simulink model "wind_model"  (R2021b)
settings: Solver=VariableStepAuto  StartTime=0.0  StopTime=500  RelTol=1e-3
values from neighbouring files (symbols this model uses):
  F = 0.0555 * (1+8*a_bar^2)*t^2*b^3    [ImIiCompute.m]
  r = 1000    [MPC.m]
undefined symbols (not defined in the file or in its folder): Light, MIL
libraries: aerolibwind2 x2, simulink x1
settings Model: Creator=zhongyuliang  LastModifiedBy=zhongyuliang

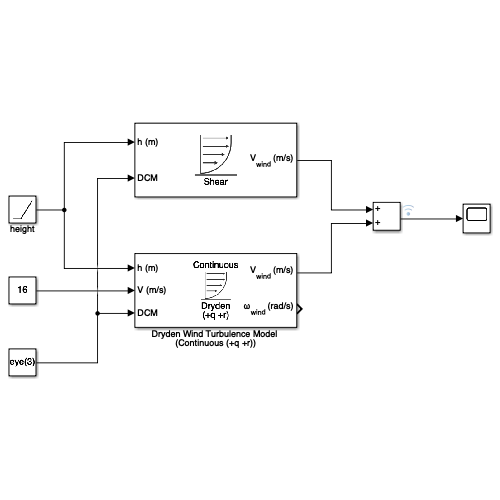
[thumbnail: Simulink's stored preview of the top-level diagram]
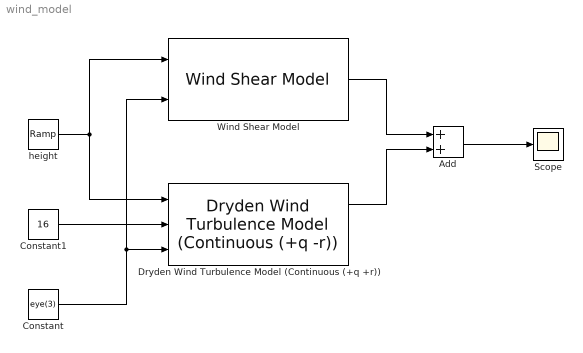
== system wind_model ==
  Add : Sum
  Constant : Constant  Value=eye(3)
  Constant1 : Constant  Value=16
  Dryden Wind Turbulence Model (Continuous (+q +r)) : aerolibwind2/Dryden Wind Turbulence Model  (Continuous (+q -r))  units=Metric (MKS)  spec=MIL-F-8785C  model=Continuous Dryden (+q +r)  W20=3  Wdeg=0  TurbProb=10^-2 - Light  L_high=533.4  Wingspan=10  ts=0.1  Seed=[23341 23342 23343 23344]  T_on=on
  Scope : Scope
  Wind Shear Model : aerolibwind2/Wind Shear Model  units=Metric (MKS)  phase=Category C - Terminal Flight Phase  W_20=15  Wdeg=0
  height : simulink/Sources/Ramp  slope=1  start=0  InitialOutput=0
  wires:
  Constant/1 -> Wind Shear Model/2, Dryden Wind Turbulence Model (Continuous (+q +r))/3
  height/1 -> Dryden Wind Turbulence Model (Continuous (+q +r))/1, Wind Shear Model/1
  Wind Shear Model/1 -> Add/1
  Constant1/1 -> Dryden Wind Turbulence Model (Continuous (+q +r))/2
  Dryden Wind Turbulence Model (Continuous (+q +r))/1 -> Add/2
  Add/1 -> Scope/1
